simulink model "three_bit_adder"  (R2021a)
settings: Solver=VariableStepAuto  StartTime=0.0  StopTime=10.0  RelTol=1e-3
settings Model: Creator=kbhar  LastModifiedBy=kbhar

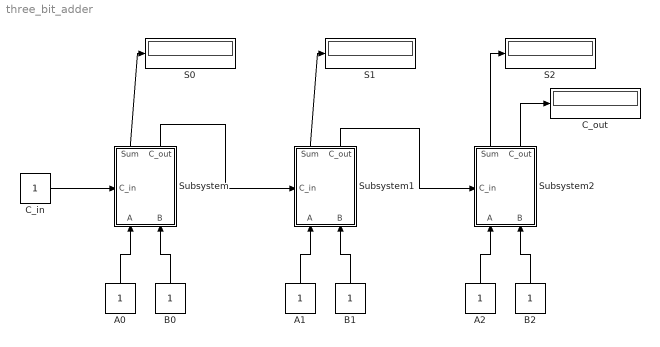
== system three_bit_adder ==
  A0 : Constant
  A1 : Constant
  A2 : Constant
  B0 : Constant
  B1 : Constant
  B2 : Constant
  C_in : Constant
  C_out : Display
  S0 : Display
  S1 : Display
  S2 : Display
  Subsystem : Subsystem
      settings: PortSchema="{\"entries\":[{\"content\":{\"sides\":[{\"content\":{\"connectorIds\":[\"In1\",\"In2\"]},\"type\":\"ConnectorPlacement.EquallySpacedRectSide\",\"uuid\":\"38d1d783-1e84-469f-b88f-34400794f458\"},{\"content\":{\"connectorIds\":[\"Out1\",\"Out2\"],\"side\":\"RIGHT\"},\"type\":\"ConnectorPlacement.EquallySpacedRectSide\",\"uuid\":\"9549b396-3b16-432f-9c12-dae7a5b8dc11\"},{\"content\":{\"connectorIds\":[\"In3\"],\"side\":\"TOP\"},\"type\":\"ConnectorPlacement.EquallySpacedRectSide\",\"uuid\":\"526a5790-86b3-4626-b4aa-b9520108ec40\"}]},\"type\":\"ConnectorPlacement.EquallySpacedConnector\",\"uuid\":\"b57ea0ad-738f-4734-9daa-a65058de1f48\"}],\"packageUris\":[\"http://schema.mathworks.com/mf0/Connector/R2020b\"],\"version\":\"1.0\"}"
  Subsystem1 : Subsystem
      settings: PortSchema="{\"entries\":[{\"content\":{\"sides\":[{\"content\":{\"connectorIds\":[\"In1\",\"In2\"]},\"type\":\"ConnectorPlacement.EquallySpacedRectSide\",\"uuid\":\"38d1d783-1e84-469f-b88f-34400794f458\"},{\"content\":{\"connectorIds\":[\"Out1\",\"Out2\"],\"side\":\"RIGHT\"},\"type\":\"ConnectorPlacement.EquallySpacedRectSide\",\"uuid\":\"9549b396-3b16-432f-9c12-dae7a5b8dc11\"},{\"content\":{\"connectorIds\":[\"In3\"],\"side\":\"TOP\"},\"type\":\"ConnectorPlacement.EquallySpacedRectSide\",\"uuid\":\"526a5790-86b3-4626-b4aa-b9520108ec40\"}]},\"type\":\"ConnectorPlacement.EquallySpacedConnector\",\"uuid\":\"b57ea0ad-738f-4734-9daa-a65058de1f48\"}],\"packageUris\":[\"http://schema.mathworks.com/mf0/Connector/R2020b\"],\"version\":\"1.0\"}"
  Subsystem2 : Subsystem
      settings: PortSchema="{\"entries\":[{\"content\":{\"sides\":[{\"content\":{\"connectorIds\":[\"In1\",\"In2\"]},\"type\":\"ConnectorPlacement.EquallySpacedRectSide\",\"uuid\":\"38d1d783-1e84-469f-b88f-34400794f458\"},{\"content\":{\"connectorIds\":[\"Out1\",\"Out2\"],\"side\":\"RIGHT\"},\"type\":\"ConnectorPlacement.EquallySpacedRectSide\",\"uuid\":\"9549b396-3b16-432f-9c12-dae7a5b8dc11\"},{\"content\":{\"connectorIds\":[\"In3\"],\"side\":\"TOP\"},\"type\":\"ConnectorPlacement.EquallySpacedRectSide\",\"uuid\":\"526a5790-86b3-4626-b4aa-b9520108ec40\"}]},\"type\":\"ConnectorPlacement.EquallySpacedConnector\",\"uuid\":\"b57ea0ad-738f-4734-9daa-a65058de1f48\"}],\"packageUris\":[\"http://schema.mathworks.com/mf0/Connector/R2020b\"],\"version\":\"1.0\"}"
  wires:
  Subsystem/2(C_out) -> Subsystem1/3(C_in)
  Subsystem1/2(C_out) -> Subsystem2/3(C_in)
  A0/1 -> Subsystem/1(A)
  B0/1 -> Subsystem/2(B)
  A1/1 -> Subsystem1/1(A)
  B1/1 -> Subsystem1/2(B)
  A2/1 -> Subsystem2/1(A)
  B2/1 -> Subsystem2/2(B)
  Subsystem/1(Sum) -> S0/1
  Subsystem2/2(C_out) -> C_out/1
  Subsystem2/1(Sum) -> S2/1
  Subsystem1/1(Sum) -> S1/1
  C_in/1 -> Subsystem/3(C_in)

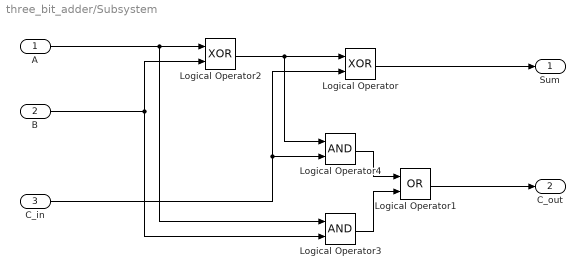
== system three_bit_adder/Subsystem ==
  A : Inport
  B : Inport  Port=2
  C_in : Inport  Port=3
  Logical Operator : Logic  Operator=XOR  AllPortsSameDT=off  OutDataTypeStr=boolean
  Logical Operator1 : Logic  Operator=OR  AllPortsSameDT=off  OutDataTypeStr=boolean
  Logical Operator2 : Logic  Operator=XOR  AllPortsSameDT=off  OutDataTypeStr=boolean
  Logical Operator3 : Logic  AllPortsSameDT=off  OutDataTypeStr=boolean
  Logical Operator4 : Logic  AllPortsSameDT=off  OutDataTypeStr=boolean
  Sum : Outport
  C_out : Outport  Port=2
  wires:
  B/1 -> Logical Operator3/2, Logical Operator2/2
  A/1 -> Logical Operator3/1, Logical Operator2/1
  Logical Operator4/1 -> Logical Operator1/1
  Logical Operator/1 -> Sum/1
  Logical Operator2/1 -> Logical Operator4/1, Logical Operator/1
  C_in/1 -> Logical Operator4/2, Logical Operator/2
  Logical Operator3/1 -> Logical Operator1/2
  Logical Operator1/1 -> C_out/1

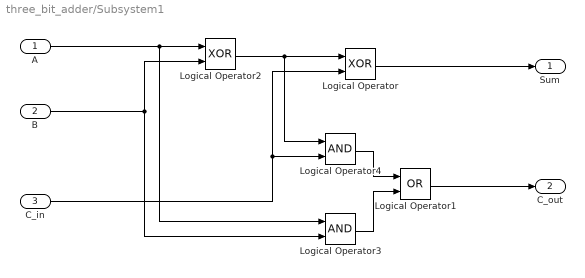
== system three_bit_adder/Subsystem1 ==
  A : Inport
  B : Inport  Port=2
  C_in : Inport  Port=3
  Logical Operator : Logic  Operator=XOR  AllPortsSameDT=off  OutDataTypeStr=boolean
  Logical Operator1 : Logic  Operator=OR  AllPortsSameDT=off  OutDataTypeStr=boolean
  Logical Operator2 : Logic  Operator=XOR  AllPortsSameDT=off  OutDataTypeStr=boolean
  Logical Operator3 : Logic  AllPortsSameDT=off  OutDataTypeStr=boolean
  Logical Operator4 : Logic  AllPortsSameDT=off  OutDataTypeStr=boolean
  Sum : Outport
  C_out : Outport  Port=2
  wires:
  B/1 -> Logical Operator3/2, Logical Operator2/2
  A/1 -> Logical Operator3/1, Logical Operator2/1
  Logical Operator4/1 -> Logical Operator1/1
  Logical Operator/1 -> Sum/1
  Logical Operator2/1 -> Logical Operator4/1, Logical Operator/1
  C_in/1 -> Logical Operator4/2, Logical Operator/2
  Logical Operator3/1 -> Logical Operator1/2
  Logical Operator1/1 -> C_out/1

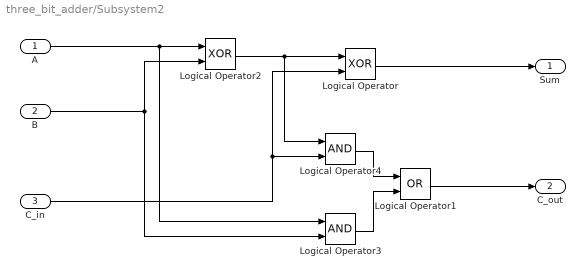
== system three_bit_adder/Subsystem2 ==
  A : Inport
  B : Inport  Port=2
  C_in : Inport  Port=3
  Logical Operator : Logic  Operator=XOR  AllPortsSameDT=off  OutDataTypeStr=boolean
  Logical Operator1 : Logic  Operator=OR  AllPortsSameDT=off  OutDataTypeStr=boolean
  Logical Operator2 : Logic  Operator=XOR  AllPortsSameDT=off  OutDataTypeStr=boolean
  Logical Operator3 : Logic  AllPortsSameDT=off  OutDataTypeStr=boolean
  Logical Operator4 : Logic  AllPortsSameDT=off  OutDataTypeStr=boolean
  Sum : Outport
  C_out : Outport  Port=2
  wires:
  B/1 -> Logical Operator3/2, Logical Operator2/2
  A/1 -> Logical Operator3/1, Logical Operator2/1
  Logical Operator4/1 -> Logical Operator1/1
  Logical Operator/1 -> Sum/1
  Logical Operator2/1 -> Logical Operator4/1, Logical Operator/1
  C_in/1 -> Logical Operator4/2, Logical Operator/2
  Logical Operator3/1 -> Logical Operator1/2
  Logical Operator1/1 -> C_out/1
